simulink library "VolumeBtc"  (R2022b)
settings: Solver=VariableStepAuto  StartTime=0.0  StopTime=10.0  RelTol=1e-3
undefined symbols (not defined in the file or in its folder): InnerLinkConfig
libraries: HandyTextFile x2, FeaturePath x1, Index2DbTableBtc x1, RTC x1, RgainyBtc x1, TuneVar x1
settings Model: Creator=st51187  LastModifiedBy=kl13806
settings SolverCC: AlgebraicLoopSolver=TrustRegion
settings DebuggingCC: UnconnectedInputMsg=warning  UnconnectedOutputMsg=warning  UnconnectedLineMsg=warning  SFMachineParentedDataDiag=warning
settings ModelReferenceCC: EnableRefExpFcnMdlSchedulingChecks=on
settings RTWCC: DLArmComputeVersion=19.05

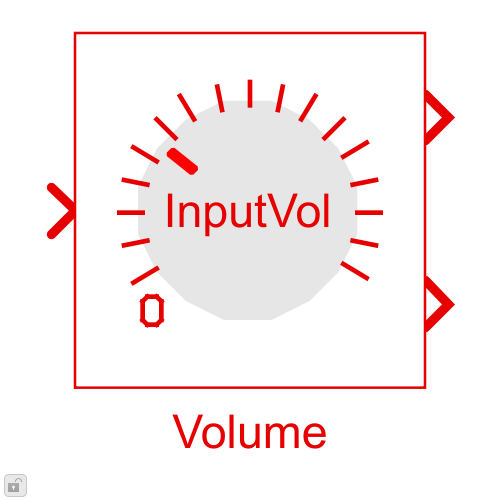
[thumbnail: Simulink's stored preview of the top-level diagram]
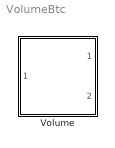
== system VolumeBtc ==
  Volume : Subsystem  mask(Blocklib Volume){FeatureName=InputVol, Config=InnerLinkConfig, EnableGainOut=on, TriggerInit=[60 35 135 110]}
      mask prompts: FeatureName "Feature path name:"; Config "VolumeConfig"; EnableGainOut "Enable gain output"; TriggerInit "Hidden: MoveFcn redraw"
      mask help: This volume signal block includes receipt of volume level (via RTC) as well as tuning variables to calibrate a gain table that maps 8-bit integer volume index (from RTC) to float decibels.
      mask init:
      | blkh=gcbh;
      | Config=BTConfig.Assert(blkh,Config);
      | 
      | % Set boundary conditions
      | rampRateBounds = [5,50000];
      | rampTimeBounds = [1,3000];
      | BTConfig.InitSetFeatureIfPresent(blkh,'FeatureName');
      | Config.Validate();
      | 
      | EnableBlockPort(blkh,'gain out',EnableGainOut);
      settings: MoveFcn=VolumeMask.CB_TriggerInit(gcbh);
      mask Help:
      | This block allows a ramped change in volume using rgainy block.
      | - The initial gain to be applied to the input audio can be set (typically 0)
      | 
      | RTC CONTROL:
      | Run time control is available to dynamically mute the audio. The volume index can be provided (typically between 0-255), along with a ramp time and rate (rate gets precedence).
      | RTC_SIM_OBJ.AddREQ( 'VolumeSet', 0.6, [0005,  <volume_index>, <ramp_db_per_second>, <ramp_time>]);
      | E.g., RTC_SIM_OBJ.AddREQ( 'VolumeSet', 0.7, [0005, 255, 0, 50]);
      mask TypeOptions FeatureName: FeaturePath/FeatureName
      mask Callback Config: BTConfig.CallbackHideIfPresent(gcbh,{'FeatureName'});
      mask Callback TriggerInit: VolumeMask.CB_TriggerInit(gcbh);
      mask Display:
      | [path,w,h] = IconVolumeMask();
      | 
      | % work in pixels since the icon does not scale
      | pos = get(gcbh,'position');
      | bw = pos(3) - pos(1);
      | bh = pos(4) - pos(2);
      | 
      | % Draw centered icon
      | xAdj = bw/2 - w/2;
      | yAdj = bh/2 - h/2;
      | for i=1:length(path)
      |     if (path(i).rgb(1) >= 0)
      |         patch(path(i).x+xAdj, path(i).y+yAdj, path(i).rgb);
      |     end
      |     if (path(i).stroke(1) >= 0)
      |         plot(path(i).x+xAdj, path(i).y+yAdj);
      |     end
      | end
      | 
      | % Display some text
      | text(bw/2, bh/2,FeatureName, ...
      |     'horizontalAlignment','center', ...
      |     'VerticalAlignment','middle');

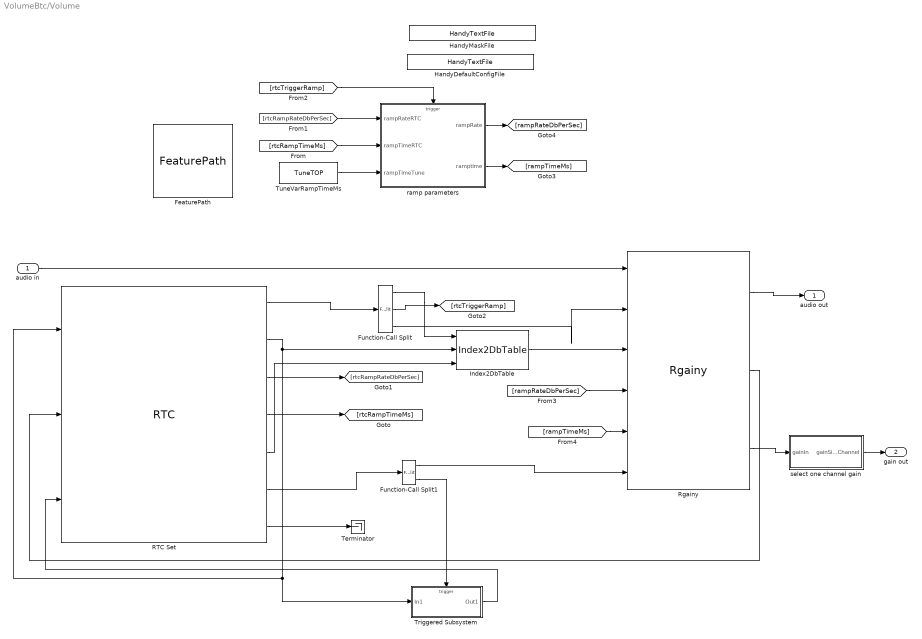
== system VolumeBtc/Volume ==
  audio in : Inport
  FeaturePath : FeaturePath/FeaturePath  FeatureName=InputVol  IsGroup=off  GroupNumber=-1  IsModule=off  TriggerInit=[640 269 755 376]
      settings: SourceProductName=Bose Talaria
  Function-Call Split : FunctionCallSplit  IconShape=distinctive  NumOutputPorts=3
  Function-Call Split1 : FunctionCallSplit  IconShape=distinctive  NumOutputPorts=2  OutputPortLayout=default
  HandyDefaultConfigFile : HandyTextFile/HandyTextFile  TemplateSource=Config  FileSuffix=Init  OpenDialogOnLoad=off  UseThisBlockName=off  TheDefaultText=|  ShowInLibBrowser=on
      | % $(FILENAME) Setup model parameters for each "Init" callback (e.g. update diagram)
      | sample_rate_in_hertz = 44100;
      | frame_size = 32;
      | sysin_channel_count = 2;
      settings: SourceProductName=Bose Talaria
  HandyMaskFile : HandyTextFile/HandyTextFile  TemplateSource=Mask  FileSuffix=Init  OpenDialogOnLoad=off  UseThisBlockName=off  TheDefaultText=|  ShowInLibBrowser=on
      | % $(FILENAME) Setup model parameters for each "Init" callback (e.g. update diagram)
      | sample_rate_in_hertz = 44100;
      | frame_size = 32;
      | sysin_channel_count = 2;
      settings: SourceProductName=Bose Talaria
  Index2DbTable : Index2DbTableBtc/Index2DbTable  Config=Config
  RTC Set : RTC/RTC  Description=|  REQ_Priority=RTC_Mask.NormalPriority  RequestAtInit=off  EnableRequest=on  REQElemName1=gain_index  REQElemType1=uint32  REQElemWidth1=1  REQElemInitial1=[]  REQElemName2=ramp_db_per_second  REQElemType2=uint32  REQElemWidth2=1  REQElemInitial2=[]  REQElemName3=ramp_milliseconds  REQElemType3=uint32  REQElemWidth3=1  REQElemInitial3=[]  REQElemName4=gain_offset  REQElemType4=int32  REQElemWidth4=1  REQElemInitial4=[]  REQElemType5=uint32  REQElemWidth5=1  REQElemInitial5=[]  REQElemType6=uint32  REQElemWidth6=1  REQElemInitial6=[]  REQElemType7=uint32  REQElemWidth7=1  REQElemInitial7=[]  REQElemType8=uint32  REQElemWidth8=1  REQElemInitial8=[]  REQElemType9=uint32  REQElemWidth9=1  REQElemInitial9=[]  REQElemType10=uint32  REQElemWidth10=1  REQElemInitial10=[]  EnableResponse=on  EnableRSP_StatusIn=off  RSPElemName1=gain_index  RSPElemType1=uint32  RSPElemWidth1=1  RSPElemType2=uint32  RSPElemWidth2=1  RSPElemType3=uint32  RSPElemWidth3=1  RSPElemType4=uint32  RSPElemWidth4=1  RSPElemType5=uint32  RSPElemWidth5=1  RSPElemType6=uint32  RSPElemWidth6=1  RSPElemType7=uint32  RSPElemWidth7=1  RSPElemType8=uint32  RSPElemWidth8=1  RSPElemType9=uint32  RSPElemWidth9=1  RSPElemType10=uint32  RSPElemWidth10=1  EnableNotification=on  EnableNTF_PrepTrig=on  NTFElemName1=gain_index  NTFElemType1=uint32  NTFElemWidth1=1  NTFElemType2=uint32  NTFElemWidth2=1  NTFElemType3=uint32  NTFElemWidth3=1  NTFElemType4=uint32  NTFElemWidth4=1  NTFElemType5=uint32  NTFElemWidth5=1  NTFElemType6=uint32  NTFElemWidth6=1  NTFElemType7=uint32  NTFElemWidth7=1  NTFElemType8=uint32  NTFElemWidth8=1  NTFElemType9=uint32  NTFElemWidth9=1  NTFElemType10=uint32  NTFElemWidth10=1  MaskMessageName=Set
      | Sets new target volume.
      | Provide the target volume as 8 bit index value to be mapped through a tunable VolumeTable.
      |  
      | To use slope-based ramping:
      | ----------------------------------
      | When db_per_second has a non-zero value,ramp_milliseconds is ignored and db_per_second controls the ramp.
      |  
      | To use time-based ramping:
      | ----------------------------------
      | The value of db_per_second must be zero for ramp milliseconds to then control the ramping.
      settings: SourceProductName=Bose Talaria
  Rgainy : RgainyBtc/Rgainy  GainOutEnable=on  Config=Config.Rgainy
  Terminator : Terminator
  Triggered Subsystem : Subsystem  TreatAsAtomicUnit=on
  TuneVarRampTimeMs : TuneVar/TuneTOP  TriggerInit=[825 324 910 356]  TopName=RampTime  TuneName=RampTime  DataType=single  TunabilityNumber=1  MinValue=[]  MaxValue=[]  BankNumber=0  PreOverlay=false  PostOverlay=false  UseSameName=on  MaskValue=100
      settings: SourceProductName=Bose Talaria
  ramp parameters : MATLAB Function  TreatAsAtomicUnit=on
  select one channel gain : MATLAB Function  TreatAsAtomicUnit=on
  audio out : Outport  VectorParamsAs1DForOutWhenUnconnected=off
  gain out : Outport  Port=2
  wires:
  Function-Call Split/1 -> Index2DbTable/1
  ramp parameters/2(ramptime) -> [rampTimeMs]
  ramp parameters/1(rampRate) -> [rampRateDbPerSec]
  [rtcTriggerRamp] -> ramp parameters/Trigger
  RTC Set/5 -> Index2DbTable/3
  [rampTimeMs] -> Rgainy/5
  RTC Set/4 -> [rtcRampTimeMs]
  [rtcRampRateDbPerSec] -> ramp parameters/1(rampRateRTC)
  Rgainy/2 -> RTC Set/2
  Rgainy/1 -> audio out/1
  audio in/1 -> Rgainy/1
  RTC Set/3 -> [rtcRampRateDbPerSec]
  Function-Call Split1/1 -> Rgainy/6
  Function-Call Split1/2 -> Triggered Subsystem/Trigger
  RTC Set/1 -> Function-Call Split/1
  RTC Set/7 -> Terminator/1
  Function-Call Split/2 -> [rtcTriggerRamp]
  RTC Set/6 -> Function-Call Split1/1
  Function-Call Split/3 -> Rgainy/2
  Index2DbTable/1 -> Rgainy/3
  [rtcRampTimeMs] -> ramp parameters/2(rampTimeRTC)
  TuneVarRampTimeMs/1 -> ramp parameters/3(rampTimeTune)
  [rampRateDbPerSec] -> Rgainy/4
  select one channel gain/1(gainSingleChannel) -> gain out/1
  Rgainy/3 -> select one channel gain/1(gainIn)
  Triggered Subsystem/1(Out1) -> RTC Set/3
  RTC Set/2 -> Triggered Subsystem/1(In1), RTC Set/1, Index2DbTable/2

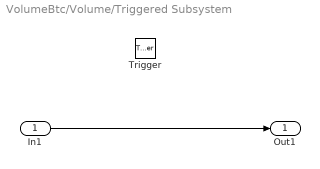
== system VolumeBtc/Volume/Triggered Subsystem ==
  In1 : Inport
  Trigger : TriggerPort  TriggerType=function-call  VariantControl=Variant
  Out1 : Outport
  wires:
  In1/1 -> Out1/1

== matlab function VolumeBtc/Volume/ramp parameters ==
  data rampRateRTC settings: description="If provided (i.e. non zero), this argument causes the \"ramp times (ms)\" input to be ignored. The block will calculate ramp times itself to ensure all gain changes happen at the db_per_sec slope provided."
  data rampTimeRTC settings: description=This vector signal must provide a linear target gain for every ramper.
  data rampTimeTune settings: description=|
      | The rampTimes_ms signal can accept one or more ramp times. If only one time is given, it is applied to all rampers. When more than one time is given, the times are delt out to the rampers in order. If not enough times are specified to cover all the rampers, the last given time is filled in to any remaining rampers.
      | NOTE: this input signal is entirely ignored if the db_per_sec input signal is non-zero. Attach the db_per_sec input to a ground block if you want to provide ramp times via this input.
  data rampTimeBounds settings: description="This input is required for control calculations to work. The \"Audio Stats\" block is a handy tool to lift this property right off an inbound audio signal and feed it to this block automatically without using workspace parameters or other constants."
  data rampRateBounds settings: description="This input is required for control calculations to work. The \"Audio Stats\" block is a handy tool to lift this property right off an inbound audio signal and feed it to this block automatically without using workspace parameters or other constants."
  data: rampRateRTC input; rampRate output; rampTimeRTC input; rampTimeTune input; ramptime output; rampTimeBounds parameter; rampRateBounds parameter
  events: trigger input FUNCTION_CALL_EVENT
function [rampRate, ramptime] = get_ramp_parameters(...
    rampRateRTC, rampTimeRTC, rampTimeTune,... % inputs
    rampTimeBounds, rampRateBounds) % parameters

% Ramp time and rate are provided to the block through RTC messages. However 
% in case neither of them are provided, the block will use the default ramp 
% time given in the tune variables.

    ramptime = single(rampTimeTune);
    rampRate = single(0);
    
    if (rampRateRTC)
        rampRate = single(rampRateRTC);
        rampRate = max(rampRateBounds(1), rampRate);
        rampRate = min(rampRateBounds(2), rampRate);
    end
    if (rampTimeRTC)
        ramptime = single(rampTimeRTC);
    end
    ramptime = max(rampTimeBounds(1), ramptime);
    ramptime = min(rampTimeBounds(2), ramptime);
end

== matlab function VolumeBtc/Volume/select one channel gain ==
  data: gainIn input; gainSingleChannel output
function gainSingleChannel = fcn(gainIn)
% Rgainy outputs gains of all channels. In the entertainment path, we only
% have one ramper meaning that the same gain gets applied to all channels.
% The following code extracts the gain of just the first channel as output.
    gainSingleChannel = squeeze(gainIn(:,1,:));
